simulink model "Revolution_Open_Loop_Frenquency_Module"  (Simulink 7.5)
settings: Solver=ode23s  StartTime=0.0  StopTime=8  RelTol=1e-3  AbsTol=1e-3
libraries: powerlib x9, powerlib_extras x3
settings Model: Creator=lm  LastModifiedBy=lm

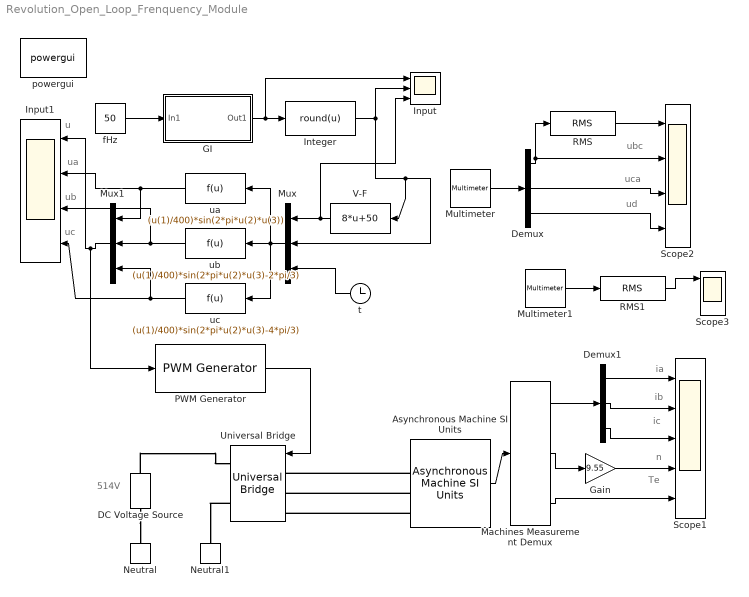
== system Revolution_Open_Loop_Frenquency_Module ==
  note: 514V
  note: ua
  note: ub
  note: uc
  note: u
  note: ubc
  note: uca
  note: ud
  note: ia
  note: ib
  note: ic
  note: n
  note: Te
  Asynchronous Machine SI Units : powerlib/Machines/Asynchronous Machine SI Units  DialogController=POWERSYS.PowerSysDialog  SystemSampleTime=-1  PresetModel="19:  100 HP (75KW)  400 V 50Hz 1484 RPM"  MechanicalLoad=Torque Tm  ShowDetailedParameters=on  RotorType=Squirrel-cage  ReferenceFrame=Rotor  NominalParameters=[7.5e+004 400 50]  Stator=[0.03552 0.000335]  Rotor=[0.02092 0.000335]  Lm=0.0151  Mechanical=[1.25 0.03914 2]  PolePairs=2  InitialConditions=[1 0 0 0 0 0 0 0]  Units=SI  LoadFlowParameters=1492000  SimulateSaturation=off  Saturation=[14.03593122, 27.81365428, 53.79336849, 72.68890987, 97.98006896, 148.6815601, 215.7428561, 302.9841135, 428.7778367 ; 230, 322, 414, 460, 506, 552, 598, 644, 690]  TsPowergui=0  TsBlock=-1  IterativeModel=Forward Euler
  DC Voltage Source : powerlib/Electrical Sources/DC Voltage Source  DialogController=POWERSYS.PowerSysDialog  SystemSampleTime=-1  Amplitude=514  Measurements=None
  Demux : Demux  Outputs=3
  Demux1 : Demux  Outputs=3
  GI : Subsystem
  Gain : Gain  Gain=9.55  ParameterDataType=fixdt(1, 16)  ParameterScaling=2^0  OutDataType=fixdt(1, 16)  OutScaling=2^0
  Input : Scope  NumInputPorts=3
      settings: YMin=27~27~265  YMax=30.5~30.5~295
  Input1 : Scope  NumInputPorts=4
      settings: TimeRange=0.8  YMin=-1~-1~-1~-1  YMax=1~1~1~1  SaveName=ScopeData2
  Integer : MATLABFcn  MATLABFcn=round(u)
  Machines Measurement Demux : powerlib/Machines/Machines Measurement Demux  DialogController=POWERSYS.PowerSysDialog  SystemSampleTime=-1  machType=Asynchronous  ssm1=on  ssm2=on  ssm3=on  ssm4=on  ssm5=on  ssm6=on  sm1=on  sm2=off  sm3=off  sm4=off  sm5=off  sm6=off  sm7=off  sm8=on  sm9=off  sm10=off  sm11=off  sm115=on  sm12=off  sm13=off  sm14=off  asm1=on  asm2=off  asm3=off  asm4=off  asm5=off  asm6=off  asm7=off  asm8=off  asm9=on  asm10=on  asm11=off  pmsm1=on  pmsm2=on  pmsm3=on  pmsm4=off  pmsm5=on  pmsm6=on  pmsm7=on  lastType=1
  Multimeter : powerlib/Measurements/Multimeter  SystemSampleTime=-1  PhasorSimulation=off  OutputType=Complex  sel=[2 3 4]  L=4  Gain=[1 1 1]  yselected={'Ubc: Universal Bridge','Uca: Universal Bridge','Udc: Universal Bridge'};  PSBOutputType=1  PSBequivalent=0  AxesSetting=[0,0.1,-100,100]  Display=0  SavedBlockNames=-11
  Multimeter1 : powerlib/Measurements/Multimeter  SystemSampleTime=-1  PhasorSimulation=off  OutputType=Complex  sel=1  L=4  Gain=1  yselected={'Uab: Universal Bridge'};  PSBOutputType=1  PSBequivalent=0  AxesSetting=[0,0.1,-100,100]  Display=0  SavedBlockNames=-11
  Mux : Mux  Inputs=3
  Mux1 : Mux  Inputs=3
  Neutral : powerlib/Elements/Neutral  DialogController=POWERSYS.PowerSysDialog  PhysicalDomain=powersysdomain  SubClassName=unknown  LeftPortType=p1  RightPortType=p1  LConnTagsString=a  NodeNumber=10
  Neutral1 : powerlib/Elements/Neutral  DialogController=POWERSYS.PowerSysDialog  PhysicalDomain=powersysdomain  SubClassName=unknown  LeftPortType=p1  RightPortType=p1  LConnTagsString=a  NodeNumber=10
  PWM Generator : powerlib_extras/Control  Blocks/PWM Generator  DialogController=POWERSYS.PowerSysDialog  SystemSampleTime=-1  GeneratorMode="3-arm  bridge (6 pulses)"  Fc=1500  Internal=off  mIndex=0.4  Freq=60  Phase=0
  RMS : powerlib_extras/Measurements/RMS  DialogController=POWERSYS.PowerSysDialog  SystemSampleTime=-1  f1=50
  RMS1 : powerlib_extras/Measurements/RMS  DialogController=POWERSYS.PowerSysDialog  SystemSampleTime=-1  f1=50
  Scope1 : Scope  NumInputPorts=5
      settings: YMin=-40~-40~-30~1600~-12.5  YMax=40~40~40~2500~7.5
  Scope2 : Scope  NumInputPorts=4
      settings: TimeRange=0.4315445026178011  YMin=0~-1.5e+184~-3.796599158636241e+054~513  YMax=3.374982646119674e+093~4.999999999999999e+183~2e+184~515  SaveName=ScopeData4
  Scope3 : Scope  NumInputPorts=4
      settings: TimeRange=0.4315445026178011  YMin=-750~-1~-1~-1  YMax=750~1~1~1  SaveName=ScopeData3
  Universal Bridge : powerlib/Power Electronics/Universal Bridge  DialogController=POWERSYS.PowerSysDialog  SystemSampleTime=-1  Arms=3  SnubberResistance=1e5  SnubberCapacitance=inf  Device=IGBT / Diodes  Ron=1e-3  Lon=0  ForwardVoltages="[  0  0  ]"  ForwardVoltage=0  GTOparameters=[ 10e-6 , 20e-6 ]  IGBTparameters=[ 1e-6 , 2e-6 ]  Measurements=UAB UBC UCA UDC voltages  Measurements_2=None  converterType=Rectifier
  V-F : Fcn  Expr=8*u+50
  fHz : Constant  Value=50  OutDataType=fixdt(1, 16)  OutScaling=2^0
  powergui : powerlib/powergui  Priority=1  SystemSampleTime=-1  SimulationMode=Discrete  SampleTime=50e-6  frequency=60  SPID=off  DisableSnubberDevices=off  DisableRonSwitches=off  DisableVfSwitches=off  SwTol=0  Interpol=off  frequencyindice=50  echomessages=off  HookPort=off  DisplayEquations=off  FunctionMessages=off  EnableUseOfTLC=off  x0status=blocks  RestoreLinks=warning  ResistiveCurrentMeasurement=off  Ylog=off  Xlog=on  ShowGrid=off  save=off  variable=ZData  ZoomFFT=off  StartTime=0.0  cycles=1  DisplayStyle=1  FreqAxis=off  MaxFrequency=1000  frequencyindicesteady=1  display=off  methode=off
  t : Clock
      settings: Decimation=10
  ua : Fcn  Expr=(u(1)/400)*sin(2*pi*u(2)*u(3))
  ub : Fcn  Expr=(u(1)/400)*sin(2*pi*u(2)*u(3)-2*pi/3)
  uc : Fcn  Expr=(u(1)/400)*sin(2*pi*u(2)*u(3)-4*pi/3)
  wires:
  PWM Generator/1 -> Universal Bridge/1
  V-F/1 -> Input/3, Mux/1
  ua/1 -> Mux1/1, Input1/2
  ub/1 -> Mux1/2, Input1/3
  uc/1 -> Mux1/3, Input1/4
  Mux1/1 -> Input1/1, PWM Generator/1
  Mux/1 -> ub/1, ua/1, uc/1
  fHz/1 -> GI/1(In1)
  GI/1(Out1) -> Input/1, Integer/1
  Asynchronous Machine SI Units/1 -> Machines Measurement Demux/1
  Machines Measurement Demux/1 -> Demux1/1
  Machines Measurement Demux/2 -> Gain/1
  Demux1/1 -> Scope1/1
  Demux1/2 -> Scope1/2
  Demux1/3 -> Scope1/3
  Gain/1 -> Scope1/4
  Machines Measurement Demux/3 -> Scope1/5
  Multimeter/1 -> Demux/1
  Demux/1 -> Scope2/2, RMS/1
  Demux/2 -> Scope2/3
  Demux/3 -> Scope2/4
  t/1 -> Mux/3
  RMS/1 -> Scope2/1
  Multimeter1/1 -> RMS1/1
  RMS1/1 -> Scope3/1
  Integer/1 -> Input/2, Mux/2, V-F/1
  connections:
  DC Voltage Source/RConn1 -- Universal Bridge/RConn1
  DC Voltage Source/LConn1 -- Neutral/LConn1
  Universal Bridge/RConn2 -- Neutral1/LConn1
  Asynchronous Machine SI Units/LConn3 -- Universal Bridge/LConn3
  Asynchronous Machine SI Units/LConn2 -- Universal Bridge/LConn2
  Asynchronous Machine SI Units/LConn1 -- Universal Bridge/LConn1

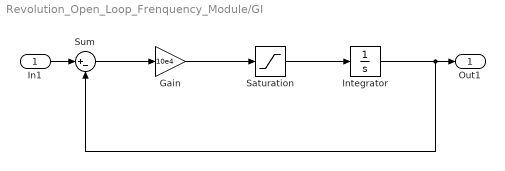
== system Revolution_Open_Loop_Frenquency_Module/GI ==
  In1 : Inport
  Gain : Gain  Gain=10e4  ParameterDataType=fixdt(1, 16)  ParameterScaling=2^0  OutDataType=fixdt(1, 16)  OutScaling=2^0
  Integrator : Integrator
  Saturation : Saturate  UpperLimit=10  LowerLimit=-10  OutDataType=fixdt(1, 16)  OutScaling=2^0
  Sum : Sum  Inputs=|+-  OutDataType=fixdt(1, 16)  OutScaling=2^0
  Out1 : Outport
  wires:
  In1/1 -> Sum/1
  Integrator/1 -> Out1/1, Sum/2
  Saturation/1 -> Integrator/1
  Gain/1 -> Saturation/1
  Sum/1 -> Gain/1
